simulink model "ctrl_custom"  (R2016b)
settings: Solver=ode3  StartTime=0.0  StopTime=inf  FixedStep=0.01  RelTol=1e-3  EnableMultiTasking=on
undefined symbols (not defined in the file): C, D, DiscIntNeverNeededParam, eps_c, epsilon, hd, hd2, I_s, k_cc, K_omega, K_q1f, K_q1r, K_q2f, K_q2r, K_q3f, K_q3r, K_q4f, K_q4r, K_q5f, K_q5r, K_q6f, K_q6r, K_T1f, K_T1r, K_T2f, K_T2r, K_T3f, K_T3r, K_T4f, K_T4r, K_T5f, K_T5r, K_T6f, K_T6r, Kp, Max_Acceleration, Max_rotation, Max_thrust, Min_thrust, n_c, n_max, p_cc, pwm_thr1_backward, pwm_thr1_forward, pwm_thr2_backward, pwm_thr2_forward, pwm_thr3_backward, pwm_thr3_forward, pwm_thr4_backward, pwm_thr4_forward, pwm_thr5_backward, pwm_thr5_forward, pwm_thr6_backward, pwm_thr6_forward, Q_f0, Q_max, r_cc, Rho, Thruster
libraries: dspmtrx3 x9, marine_gnc x9, simulink x7, simulink_extras x3
(part 3 of 6)

== system ctrl_custom/Initialization of parameters/Control Gains ==
  Create Diagonal Matrix : dspmtrx3/Create Diagonal Matrix
  Create Diagonal Matrix1 : dspmtrx3/Create Diagonal Matrix
  Create Diagonal Matrix2 : dspmtrx3/Create Diagonal Matrix
  K_d_psi : S-Function  Priority=7  FunctionName=NIVeriStandIO  Parameters=width dtype portnum stime stype btype  SFunctionDeploymentMode=off  EnableBusSupport=off  mask(NI VeriStand Inport){portnum=7, width=-1, stime=-1, dtype=auto, stype=auto, btype=1}
      mask prompts: portnum "Port number:"; width "Port dimensions (-1 for dynamically sized):"; stime "Sample time (-1 for inherited):"; dtype "Data type:"; stype "Signal type:"; btype "Block type:"
      mask help: Use this inport on any level of nested subsystems to allow NI VeriStand software to map signals to it.
      mask init:
      | NIVeriStandIO_init;
      settings: CopyFcn=NIVeriStand_MDL_functions('', 'IO_copy');  DeleteFcn=NIVeriStand_MDL_functions('', 'IO_delete');  MoveFcn=set_param(gcb, 'Mask', 'on');
      mask Callback portnum: NIVeriStand_MDL_functions('', 'IO_setportnum');
      mask TypeOptions dtype: auto | double | single | int8 | uint8 | int16 | uint16 | int32 | uint32 | boolean
      mask Callback dtype: NIVeriStand_MDL_functions('', 'IO_booleansignal');
      mask TypeOptions stype: auto | real | complex
      mask Display:
      | patch([-x x], [-y y], [.90980 .81960 .32156]);
      | plot([xrad -x x xrad], [yrad -y y yrad]);
      | fprintf('NI In%d', portnum);
  K_d_x : S-Function  Priority=8  FunctionName=NIVeriStandIO  Parameters=width dtype portnum stime stype btype  SFunctionDeploymentMode=off  EnableBusSupport=off  mask(NI VeriStand Inport){portnum=8, width=-1, stime=-1, dtype=auto, stype=auto, btype=1}
      mask prompts: portnum "Port number:"; width "Port dimensions (-1 for dynamically sized):"; stime "Sample time (-1 for inherited):"; dtype "Data type:"; stype "Signal type:"; btype "Block type:"
      mask help: Use this inport on any level of nested subsystems to allow NI VeriStand software to map signals to it.
      mask init:
      | NIVeriStandIO_init;
      settings: CopyFcn=NIVeriStand_MDL_functions('', 'IO_copy');  DeleteFcn=NIVeriStand_MDL_functions('', 'IO_delete');  MoveFcn=set_param(gcb, 'Mask', 'on');
      mask Callback portnum: NIVeriStand_MDL_functions('', 'IO_setportnum');
      mask TypeOptions dtype: auto | double | single | int8 | uint8 | int16 | uint16 | int32 | uint32 | boolean
      mask Callback dtype: NIVeriStand_MDL_functions('', 'IO_booleansignal');
      mask TypeOptions stype: auto | real | complex
      mask Display:
      | patch([-x x], [-y y], [.90980 .81960 .32156]);
      | plot([xrad -x x xrad], [yrad -y y yrad]);
      | fprintf('NI In%d', portnum);
  K_d_y : S-Function  Priority=9  FunctionName=NIVeriStandIO  Parameters=width dtype portnum stime stype btype  SFunctionDeploymentMode=off  EnableBusSupport=off  mask(NI VeriStand Inport){portnum=9, width=-1, stime=-1, dtype=auto, stype=auto, btype=1}
      mask prompts: portnum "Port number:"; width "Port dimensions (-1 for dynamically sized):"; stime "Sample time (-1 for inherited):"; dtype "Data type:"; stype "Signal type:"; btype "Block type:"
      mask help: Use this inport on any level of nested subsystems to allow NI VeriStand software to map signals to it.
      mask init:
      | NIVeriStandIO_init;
      settings: CopyFcn=NIVeriStand_MDL_functions('', 'IO_copy');  DeleteFcn=NIVeriStand_MDL_functions('', 'IO_delete');  MoveFcn=set_param(gcb, 'Mask', 'on');
      mask Callback portnum: NIVeriStand_MDL_functions('', 'IO_setportnum');
      mask TypeOptions dtype: auto | double | single | int8 | uint8 | int16 | uint16 | int32 | uint32 | boolean
      mask Callback dtype: NIVeriStand_MDL_functions('', 'IO_booleansignal');
      mask TypeOptions stype: auto | real | complex
      mask Display:
      | patch([-x x], [-y y], [.90980 .81960 .32156]);
      | plot([xrad -x x xrad], [yrad -y y yrad]);
      | fprintf('NI In%d', portnum);
  K_i_psi : S-Function  Priority=4  FunctionName=NIVeriStandIO  Parameters=width dtype portnum stime stype btype  SFunctionDeploymentMode=off  EnableBusSupport=off  mask(NI VeriStand Inport){portnum=4, width=-1, stime=-1, dtype=auto, stype=auto, btype=1}
      mask prompts: portnum "Port number:"; width "Port dimensions (-1 for dynamically sized):"; stime "Sample time (-1 for inherited):"; dtype "Data type:"; stype "Signal type:"; btype "Block type:"
      mask help: Use this inport on any level of nested subsystems to allow NI VeriStand software to map signals to it.
      mask init:
      | NIVeriStandIO_init;
      settings: CopyFcn=NIVeriStand_MDL_functions('', 'IO_copy');  DeleteFcn=NIVeriStand_MDL_functions('', 'IO_delete');  MoveFcn=set_param(gcb, 'Mask', 'on');
      mask Callback portnum: NIVeriStand_MDL_functions('', 'IO_setportnum');
      mask TypeOptions dtype: auto | double | single | int8 | uint8 | int16 | uint16 | int32 | uint32 | boolean
      mask Callback dtype: NIVeriStand_MDL_functions('', 'IO_booleansignal');
      mask TypeOptions stype: auto | real | complex
      mask Display:
      | patch([-x x], [-y y], [.90980 .81960 .32156]);
      | plot([xrad -x x xrad], [yrad -y y yrad]);
      | fprintf('NI In%d', portnum);
  K_i_x : S-Function  Priority=5  FunctionName=NIVeriStandIO  Parameters=width dtype portnum stime stype btype  SFunctionDeploymentMode=off  EnableBusSupport=off  mask(NI VeriStand Inport){portnum=5, width=-1, stime=-1, dtype=auto, stype=auto, btype=1}
      mask prompts: portnum "Port number:"; width "Port dimensions (-1 for dynamically sized):"; stime "Sample time (-1 for inherited):"; dtype "Data type:"; stype "Signal type:"; btype "Block type:"
      mask help: Use this inport on any level of nested subsystems to allow NI VeriStand software to map signals to it.
      mask init:
      | NIVeriStandIO_init;
      settings: CopyFcn=NIVeriStand_MDL_functions('', 'IO_copy');  DeleteFcn=NIVeriStand_MDL_functions('', 'IO_delete');  MoveFcn=set_param(gcb, 'Mask', 'on');
      mask Callback portnum: NIVeriStand_MDL_functions('', 'IO_setportnum');
      mask TypeOptions dtype: auto | double | single | int8 | uint8 | int16 | uint16 | int32 | uint32 | boolean
      mask Callback dtype: NIVeriStand_MDL_functions('', 'IO_booleansignal');
      mask TypeOptions stype: auto | real | complex
      mask Display:
      | patch([-x x], [-y y], [.90980 .81960 .32156]);
      | plot([xrad -x x xrad], [yrad -y y yrad]);
      | fprintf('NI In%d', portnum);
  K_i_y : S-Function  Priority=6  FunctionName=NIVeriStandIO  Parameters=width dtype portnum stime stype btype  SFunctionDeploymentMode=off  EnableBusSupport=off  mask(NI VeriStand Inport){portnum=6, width=-1, stime=-1, dtype=auto, stype=auto, btype=1}
      mask prompts: portnum "Port number:"; width "Port dimensions (-1 for dynamically sized):"; stime "Sample time (-1 for inherited):"; dtype "Data type:"; stype "Signal type:"; btype "Block type:"
      mask help: Use this inport on any level of nested subsystems to allow NI VeriStand software to map signals to it.
      mask init:
      | NIVeriStandIO_init;
      settings: CopyFcn=NIVeriStand_MDL_functions('', 'IO_copy');  DeleteFcn=NIVeriStand_MDL_functions('', 'IO_delete');  MoveFcn=set_param(gcb, 'Mask', 'on');
      mask Callback portnum: NIVeriStand_MDL_functions('', 'IO_setportnum');
      mask TypeOptions dtype: auto | double | single | int8 | uint8 | int16 | uint16 | int32 | uint32 | boolean
      mask Callback dtype: NIVeriStand_MDL_functions('', 'IO_booleansignal');
      mask TypeOptions stype: auto | real | complex
      mask Display:
      | patch([-x x], [-y y], [.90980 .81960 .32156]);
      | plot([xrad -x x xrad], [yrad -y y yrad]);
      | fprintf('NI In%d', portnum);
  K_p_psi : S-Function  Priority=3  FunctionName=NIVeriStandIO  Parameters=width dtype portnum stime stype btype  SFunctionDeploymentMode=off  EnableBusSupport=off  mask(NI VeriStand Inport){portnum=3, width=-1, stime=-1, dtype=auto, stype=auto, btype=1}
      mask prompts: portnum "Port number:"; width "Port dimensions (-1 for dynamically sized):"; stime "Sample time (-1 for inherited):"; dtype "Data type:"; stype "Signal type:"; btype "Block type:"
      mask help: Use this inport on any level of nested subsystems to allow NI VeriStand software to map signals to it.
      mask init:
      | NIVeriStandIO_init;
      settings: CopyFcn=NIVeriStand_MDL_functions('', 'IO_copy');  DeleteFcn=NIVeriStand_MDL_functions('', 'IO_delete');  MoveFcn=set_param(gcb, 'Mask', 'on');
      mask Callback portnum: NIVeriStand_MDL_functions('', 'IO_setportnum');
      mask TypeOptions dtype: auto | double | single | int8 | uint8 | int16 | uint16 | int32 | uint32 | boolean
      mask Callback dtype: NIVeriStand_MDL_functions('', 'IO_booleansignal');
      mask TypeOptions stype: auto | real | complex
      mask Display:
      | patch([-x x], [-y y], [.90980 .81960 .32156]);
      | plot([xrad -x x xrad], [yrad -y y yrad]);
      | fprintf('NI In%d', portnum);
  K_p_x : S-Function  Priority=1  FunctionName=NIVeriStandIO  Parameters=width dtype portnum stime stype btype  SFunctionDeploymentMode=off  EnableBusSupport=off  mask(NI VeriStand Inport){portnum=1, width=-1, stime=-1, dtype=auto, stype=auto, btype=1}
      mask prompts: portnum "Port number:"; width "Port dimensions (-1 for dynamically sized):"; stime "Sample time (-1 for inherited):"; dtype "Data type:"; stype "Signal type:"; btype "Block type:"
      mask help: Use this inport on any level of nested subsystems to allow NI VeriStand software to map signals to it.
      mask init:
      | NIVeriStandIO_init;
      settings: CopyFcn=NIVeriStand_MDL_functions('', 'IO_copy');  DeleteFcn=NIVeriStand_MDL_functions('', 'IO_delete');  MoveFcn=set_param(gcb, 'Mask', 'on');
      mask Callback portnum: NIVeriStand_MDL_functions('', 'IO_setportnum');
      mask TypeOptions dtype: auto | double | single | int8 | uint8 | int16 | uint16 | int32 | uint32 | boolean
      mask Callback dtype: NIVeriStand_MDL_functions('', 'IO_booleansignal');
      mask TypeOptions stype: auto | real | complex
      mask Display:
      | patch([-x x], [-y y], [.90980 .81960 .32156]);
      | plot([xrad -x x xrad], [yrad -y y yrad]);
      | fprintf('NI In%d', portnum);
  K_p_y : S-Function  Priority=2  FunctionName=NIVeriStandIO  Parameters=width dtype portnum stime stype btype  SFunctionDeploymentMode=off  EnableBusSupport=off  mask(NI VeriStand Inport){portnum=2, width=-1, stime=-1, dtype=auto, stype=auto, btype=1}
      mask prompts: portnum "Port number:"; width "Port dimensions (-1 for dynamically sized):"; stime "Sample time (-1 for inherited):"; dtype "Data type:"; stype "Signal type:"; btype "Block type:"
      mask help: Use this inport on any level of nested subsystems to allow NI VeriStand software to map signals to it.
      mask init:
      | NIVeriStandIO_init;
      settings: CopyFcn=NIVeriStand_MDL_functions('', 'IO_copy');  DeleteFcn=NIVeriStand_MDL_functions('', 'IO_delete');  MoveFcn=set_param(gcb, 'Mask', 'on');
      mask Callback portnum: NIVeriStand_MDL_functions('', 'IO_setportnum');
      mask TypeOptions dtype: auto | double | single | int8 | uint8 | int16 | uint16 | int32 | uint32 | boolean
      mask Callback dtype: NIVeriStand_MDL_functions('', 'IO_booleansignal');
      mask TypeOptions stype: auto | real | complex
      mask Display:
      | patch([-x x], [-y y], [.90980 .81960 .32156]);
      | plot([xrad -x x xrad], [yrad -y y yrad]);
      | fprintf('NI In%d', portnum);
  Mux1 : Mux  Inputs=3
  Mux2 : Mux  Inputs=3
  Mux3 : Mux  Inputs=3
  tag scope: K_d=global, K_i=global, K_p=global, Kd_psi=global, Ki_psi=global, Kp_psi=global
  wires:
  K_p_x/1 -> Mux1/1
  K_p_psi/1 -> [Kp_psi], Mux1/3
  K_p_y/1 -> Mux1/2
  Mux1/1 -> Create Diagonal Matrix/1
  Create Diagonal Matrix/1 -> [K_p]
  Mux2/1 -> Create Diagonal Matrix1/1
  K_d_x/1 -> Mux3/1
  K_d_psi/1 -> [Kd_psi], Mux3/3
  K_d_y/1 -> Mux3/2
  Mux3/1 -> Create Diagonal Matrix2/1
  Create Diagonal Matrix1/1 -> [K_i]
  Create Diagonal Matrix2/1 -> [K_d]
  K_i_x/1 -> Mux2/1
  K_i_y/1 -> Mux2/2
  K_i_psi/1 -> [Ki_psi], Mux2/3

== system ctrl_custom/Initialization of parameters/Guidance Gains ==
  Create Diagonal Matrix3 : dspmtrx3/Create Diagonal Matrix
  Create Diagonal Matrix4 : dspmtrx3/Create Diagonal Matrix
  Create Diagonal Matrix5 : dspmtrx3/Create Diagonal Matrix
  MATLAB Function : MATLAB Function  TreatAsAtomicUnit=on
  MATLAB Function1 : MATLAB Function  TreatAsAtomicUnit=on
  MATLAB Function2 : MATLAB Function  TreatAsAtomicUnit=on
  Mux3 : Mux  Inputs=3
  Mux4 : Mux  Inputs=3
  Mux5 : Mux  Inputs=3
  T_psi : S-Function  Priority=7  FunctionName=NIVeriStandIO  Parameters=width dtype portnum stime stype btype  SFunctionDeploymentMode=off  EnableBusSupport=off  mask(NI VeriStand Inport){portnum=7, width=-1, stime=-1, dtype=auto, stype=auto, btype=1}
      mask prompts: portnum "Port number:"; width "Port dimensions (-1 for dynamically sized):"; stime "Sample time (-1 for inherited):"; dtype "Data type:"; stype "Signal type:"; btype "Block type:"
      mask help: Use this inport on any level of nested subsystems to allow NI VeriStand software to map signals to it.
      mask init:
      | NIVeriStandIO_init;
      settings: CopyFcn=NIVeriStand_MDL_functions('', 'IO_copy');  DeleteFcn=NIVeriStand_MDL_functions('', 'IO_delete');  MoveFcn=set_param(gcb, 'Mask', 'on');
      mask Callback portnum: NIVeriStand_MDL_functions('', 'IO_setportnum');
      mask TypeOptions dtype: auto | double | single | int8 | uint8 | int16 | uint16 | int32 | uint32 | boolean
      mask Callback dtype: NIVeriStand_MDL_functions('', 'IO_booleansignal');
      mask TypeOptions stype: auto | real | complex
      mask Display:
      | patch([-x x], [-y y], [.90980 .81960 .32156]);
      | plot([xrad -x x xrad], [yrad -y y yrad]);
      | fprintf('NI In%d', portnum);
  T_x : S-Function  Priority=8  FunctionName=NIVeriStandIO  Parameters=width dtype portnum stime stype btype  SFunctionDeploymentMode=off  EnableBusSupport=off  mask(NI VeriStand Inport){portnum=8, width=-1, stime=-1, dtype=auto, stype=auto, btype=1}
      mask prompts: portnum "Port number:"; width "Port dimensions (-1 for dynamically sized):"; stime "Sample time (-1 for inherited):"; dtype "Data type:"; stype "Signal type:"; btype "Block type:"
      mask help: Use this inport on any level of nested subsystems to allow NI VeriStand software to map signals to it.
      mask init:
      | NIVeriStandIO_init;
      settings: CopyFcn=NIVeriStand_MDL_functions('', 'IO_copy');  DeleteFcn=NIVeriStand_MDL_functions('', 'IO_delete');  MoveFcn=set_param(gcb, 'Mask', 'on');
      mask Callback portnum: NIVeriStand_MDL_functions('', 'IO_setportnum');
      mask TypeOptions dtype: auto | double | single | int8 | uint8 | int16 | uint16 | int32 | uint32 | boolean
      mask Callback dtype: NIVeriStand_MDL_functions('', 'IO_booleansignal');
      mask TypeOptions stype: auto | real | complex
      mask Display:
      | patch([-x x], [-y y], [.90980 .81960 .32156]);
      | plot([xrad -x x xrad], [yrad -y y yrad]);
      | fprintf('NI In%d', portnum);
  T_y : S-Function  Priority=9  FunctionName=NIVeriStandIO  Parameters=width dtype portnum stime stype btype  SFunctionDeploymentMode=off  EnableBusSupport=off  mask(NI VeriStand Inport){portnum=9, width=-1, stime=-1, dtype=auto, stype=auto, btype=1}
      mask prompts: portnum "Port number:"; width "Port dimensions (-1 for dynamically sized):"; stime "Sample time (-1 for inherited):"; dtype "Data type:"; stype "Signal type:"; btype "Block type:"
      mask help: Use this inport on any level of nested subsystems to allow NI VeriStand software to map signals to it.
      mask init:
      | NIVeriStandIO_init;
      settings: CopyFcn=NIVeriStand_MDL_functions('', 'IO_copy');  DeleteFcn=NIVeriStand_MDL_functions('', 'IO_delete');  MoveFcn=set_param(gcb, 'Mask', 'on');
      mask Callback portnum: NIVeriStand_MDL_functions('', 'IO_setportnum');
      mask TypeOptions dtype: auto | double | single | int8 | uint8 | int16 | uint16 | int32 | uint32 | boolean
      mask Callback dtype: NIVeriStand_MDL_functions('', 'IO_booleansignal');
      mask TypeOptions stype: auto | real | complex
      mask Display:
      | patch([-x x], [-y y], [.90980 .81960 .32156]);
      | plot([xrad -x x xrad], [yrad -y y yrad]);
      | fprintf('NI In%d', portnum);
  w_psi : S-Function  Priority=3  FunctionName=NIVeriStandIO  Parameters=width dtype portnum stime stype btype  SFunctionDeploymentMode=off  EnableBusSupport=off  mask(NI VeriStand Inport){portnum=3, width=-1, stime=-1, dtype=auto, stype=auto, btype=1}
      mask prompts: portnum "Port number:"; width "Port dimensions (-1 for dynamically sized):"; stime "Sample time (-1 for inherited):"; dtype "Data type:"; stype "Signal type:"; btype "Block type:"
      mask help: Use this inport on any level of nested subsystems to allow NI VeriStand software to map signals to it.
      mask init:
      | NIVeriStandIO_init;
      settings: CopyFcn=NIVeriStand_MDL_functions('', 'IO_copy');  DeleteFcn=NIVeriStand_MDL_functions('', 'IO_delete');  MoveFcn=set_param(gcb, 'Mask', 'on');
      mask Callback portnum: NIVeriStand_MDL_functions('', 'IO_setportnum');
      mask TypeOptions dtype: auto | double | single | int8 | uint8 | int16 | uint16 | int32 | uint32 | boolean
      mask Callback dtype: NIVeriStand_MDL_functions('', 'IO_booleansignal');
      mask TypeOptions stype: auto | real | complex
      mask Display:
      | patch([-x x], [-y y], [.90980 .81960 .32156]);
      | plot([xrad -x x xrad], [yrad -y y yrad]);
      | fprintf('NI In%d', portnum);
  w_x : S-Function  Priority=1  FunctionName=NIVeriStandIO  Parameters=width dtype portnum stime stype btype  SFunctionDeploymentMode=off  EnableBusSupport=off  mask(NI VeriStand Inport){portnum=1, width=-1, stime=-1, dtype=auto, stype=auto, btype=1}
      mask prompts: portnum "Port number:"; width "Port dimensions (-1 for dynamically sized):"; stime "Sample time (-1 for inherited):"; dtype "Data type:"; stype "Signal type:"; btype "Block type:"
      mask help: Use this inport on any level of nested subsystems to allow NI VeriStand software to map signals to it.
      mask init:
      | NIVeriStandIO_init;
      settings: CopyFcn=NIVeriStand_MDL_functions('', 'IO_copy');  DeleteFcn=NIVeriStand_MDL_functions('', 'IO_delete');  MoveFcn=set_param(gcb, 'Mask', 'on');
      mask Callback portnum: NIVeriStand_MDL_functions('', 'IO_setportnum');
      mask TypeOptions dtype: auto | double | single | int8 | uint8 | int16 | uint16 | int32 | uint32 | boolean
      mask Callback dtype: NIVeriStand_MDL_functions('', 'IO_booleansignal');
      mask TypeOptions stype: auto | real | complex
      mask Display:
      | patch([-x x], [-y y], [.90980 .81960 .32156]);
      | plot([xrad -x x xrad], [yrad -y y yrad]);
      | fprintf('NI In%d', portnum);
  w_y : S-Function  Priority=2  FunctionName=NIVeriStandIO  Parameters=width dtype portnum stime stype btype  SFunctionDeploymentMode=off  EnableBusSupport=off  mask(NI VeriStand Inport){portnum=2, width=-1, stime=-1, dtype=auto, stype=auto, btype=1}
      mask prompts: portnum "Port number:"; width "Port dimensions (-1 for dynamically sized):"; stime "Sample time (-1 for inherited):"; dtype "Data type:"; stype "Signal type:"; btype "Block type:"
      mask help: Use this inport on any level of nested subsystems to allow NI VeriStand software to map signals to it.
      mask init:
      | NIVeriStandIO_init;
      settings: CopyFcn=NIVeriStand_MDL_functions('', 'IO_copy');  DeleteFcn=NIVeriStand_MDL_functions('', 'IO_delete');  MoveFcn=set_param(gcb, 'Mask', 'on');
      mask Callback portnum: NIVeriStand_MDL_functions('', 'IO_setportnum');
      mask TypeOptions dtype: auto | double | single | int8 | uint8 | int16 | uint16 | int32 | uint32 | boolean
      mask Callback dtype: NIVeriStand_MDL_functions('', 'IO_booleansignal');
      mask TypeOptions stype: auto | real | complex
      mask Display:
      | patch([-x x], [-y y], [.90980 .81960 .32156]);
      | plot([xrad -x x xrad], [yrad -y y yrad]);
      | fprintf('NI In%d', portnum);
  zeta_psi : S-Function  Priority=4  FunctionName=NIVeriStandIO  Parameters=width dtype portnum stime stype btype  SFunctionDeploymentMode=off  EnableBusSupport=off  mask(NI VeriStand Inport){portnum=4, width=-1, stime=-1, dtype=auto, stype=auto, btype=1}
      mask prompts: portnum "Port number:"; width "Port dimensions (-1 for dynamically sized):"; stime "Sample time (-1 for inherited):"; dtype "Data type:"; stype "Signal type:"; btype "Block type:"
      mask help: Use this inport on any level of nested subsystems to allow NI VeriStand software to map signals to it.
      mask init:
      | NIVeriStandIO_init;
      settings: CopyFcn=NIVeriStand_MDL_functions('', 'IO_copy');  DeleteFcn=NIVeriStand_MDL_functions('', 'IO_delete');  MoveFcn=set_param(gcb, 'Mask', 'on');
      mask Callback portnum: NIVeriStand_MDL_functions('', 'IO_setportnum');
      mask TypeOptions dtype: auto | double | single | int8 | uint8 | int16 | uint16 | int32 | uint32 | boolean
      mask Callback dtype: NIVeriStand_MDL_functions('', 'IO_booleansignal');
      mask TypeOptions stype: auto | real | complex
      mask Display:
      | patch([-x x], [-y y], [.90980 .81960 .32156]);
      | plot([xrad -x x xrad], [yrad -y y yrad]);
      | fprintf('NI In%d', portnum);
  zeta_x : S-Function  Priority=5  FunctionName=NIVeriStandIO  Parameters=width dtype portnum stime stype btype  SFunctionDeploymentMode=off  EnableBusSupport=off  mask(NI VeriStand Inport){portnum=5, width=-1, stime=-1, dtype=auto, stype=auto, btype=1}
      mask prompts: portnum "Port number:"; width "Port dimensions (-1 for dynamically sized):"; stime "Sample time (-1 for inherited):"; dtype "Data type:"; stype "Signal type:"; btype "Block type:"
      mask help: Use this inport on any level of nested subsystems to allow NI VeriStand software to map signals to it.
      mask init:
      | NIVeriStandIO_init;
      settings: CopyFcn=NIVeriStand_MDL_functions('', 'IO_copy');  DeleteFcn=NIVeriStand_MDL_functions('', 'IO_delete');  MoveFcn=set_param(gcb, 'Mask', 'on');
      mask Callback portnum: NIVeriStand_MDL_functions('', 'IO_setportnum');
      mask TypeOptions dtype: auto | double | single | int8 | uint8 | int16 | uint16 | int32 | uint32 | boolean
      mask Callback dtype: NIVeriStand_MDL_functions('', 'IO_booleansignal');
      mask TypeOptions stype: auto | real | complex
      mask Display:
      | patch([-x x], [-y y], [.90980 .81960 .32156]);
      | plot([xrad -x x xrad], [yrad -y y yrad]);
      | fprintf('NI In%d', portnum);
  zeta_y : S-Function  Priority=6  FunctionName=NIVeriStandIO  Parameters=width dtype portnum stime stype btype  SFunctionDeploymentMode=off  EnableBusSupport=off  mask(NI VeriStand Inport){portnum=6, width=-1, stime=-1, dtype=auto, stype=auto, btype=1}
      mask prompts: portnum "Port number:"; width "Port dimensions (-1 for dynamically sized):"; stime "Sample time (-1 for inherited):"; dtype "Data type:"; stype "Signal type:"; btype "Block type:"
      mask help: Use this inport on any level of nested subsystems to allow NI VeriStand software to map signals to it.
      mask init:
      | NIVeriStandIO_init;
      settings: CopyFcn=NIVeriStand_MDL_functions('', 'IO_copy');  DeleteFcn=NIVeriStand_MDL_functions('', 'IO_delete');  MoveFcn=set_param(gcb, 'Mask', 'on');
      mask Callback portnum: NIVeriStand_MDL_functions('', 'IO_setportnum');
      mask TypeOptions dtype: auto | double | single | int8 | uint8 | int16 | uint16 | int32 | uint32 | boolean
      mask Callback dtype: NIVeriStand_MDL_functions('', 'IO_booleansignal');
      mask TypeOptions stype: auto | real | complex
      mask Display:
      | patch([-x x], [-y y], [.90980 .81960 .32156]);
      | plot([xrad -x x xrad], [yrad -y y yrad]);
      | fprintf('NI In%d', portnum);
  tag scope: Af=global, omega=global, zeta=global
  wires:
  w_x/1 -> Mux3/1
  w_psi/1 -> Mux3/3
  w_y/1 -> Mux3/2
  Mux3/1 -> Create Diagonal Matrix3/1
  Create Diagonal Matrix3/1 -> [omega]
  Mux4/1 -> Create Diagonal Matrix4/1
  T_x/1 -> MATLAB Function/1(T_x)
  T_psi/1 -> MATLAB Function2/1(T_psi)
  T_y/1 -> MATLAB Function1/1(T_y)
  Mux5/1 -> Create Diagonal Matrix5/1
  Create Diagonal Matrix4/1 -> [zeta]
  Create Diagonal Matrix5/1 -> [Af]
  zeta_x/1 -> Mux4/1
  zeta_y/1 -> Mux4/2
  zeta_psi/1 -> Mux4/3
  MATLAB Function/1(y) -> Mux5/1
  MATLAB Function1/1(y) -> Mux5/2
  MATLAB Function2/1(y) -> Mux5/3

== system ctrl_custom/Initialization of parameters/Observer Gains ==
  Constant : Constant  Value=50
  Constant1 : Constant  Value=50
  Constant2 : Constant  Value=50
  Constant{3..8} (6 alike) : Constant
  Create Diagonal Matrix : dspmtrx3/Create Diagonal Matrix
  Create Diagonal Matrix1 : dspmtrx3/Create Diagonal Matrix
  Create Diagonal Matrix2 : dspmtrx3/Create Diagonal Matrix
  Mux1 : Mux  Inputs=3
  Mux2 : Mux  Inputs=3
  Mux3 : Mux  Inputs=3
  tag scope: K_2=global, K_3=global, K_4=global
  wires:
  Constant/1 -> Mux1/1
  Constant2/1 -> Mux1/3
  Constant1/1 -> Mux1/2
  Mux1/1 -> Create Diagonal Matrix/1
  Create Diagonal Matrix/1 -> [K_2]
  Constant3/1 -> Mux2/1
  Constant5/1 -> Mux2/3
  Constant4/1 -> Mux2/2
  Mux2/1 -> Create Diagonal Matrix1/1
  Constant8/1 -> Mux3/3
  Constant7/1 -> Mux3/2
  Mux3/1 -> Create Diagonal Matrix2/1
  Create Diagonal Matrix1/1 -> [K_3]
  Create Diagonal Matrix2/1 -> [K_4]
  Constant6/1 -> Mux3/1

== system ctrl_custom/Nonlinear Passisve Observer/Transpose Rotation Matrix ==
  psi : Inport
  y_tilde : Inport  Port=2
  Mux : Mux  Inputs=2
  Mux1 : Mux  Inputs=3
  Row1 : Fcn  Expr=cos(u(1))*u(2)+sin(u(1))*u(3)
  Row2 : Fcn  Expr=-sin(u(1))*u(2)+cos(u(1))*u(3)
  Row3 : Fcn  Expr=u(4)
  R(psi)'*y_tilde : Outport
  wires:
  Mux/1 -> Row3/1, Row2/1, Row1/1
  Row1/1 -> Mux1/1
  Row2/1 -> Mux1/2
  Row3/1 -> Mux1/3
  Mux1/1 -> R(psi)'*y_tilde/1
  psi/1 -> Mux/1
  y_tilde/1 -> Mux/2

== system ctrl_custom/Nonlinear Passisve Observer/Transpose Rotation matrix ==
  psi : Inport
  b_hat : Inport  Port=2
  Mux : Mux  Inputs=2
  Mux1 : Mux  Inputs=3
  Row1 : Fcn  Expr=cos(u(1))*u(2)+sin(u(1))*u(3)
  Row2 : Fcn  Expr=-sin(u(1))*u(2)+cos(u(1))*u(3)
  Row3 : Fcn  Expr=u(4)
  R(psi)'*b_hat : Outport
  wires:
  Mux/1 -> Row3/1, Row2/1, Row1/1
  Row1/1 -> Mux1/1
  Row2/1 -> Mux1/2
  Row3/1 -> Mux1/3
  Mux1/1 -> R(psi)'*b_hat/1
  psi/1 -> Mux/1
  b_hat/1 -> Mux/2

== system ctrl_custom/Observer output /b_hat output ==
  b_hat : Inport
  Demux : Demux  Outputs=3
  b_psi_hat : S-Function  Priority=3  FunctionName=NIVeriStandIO  Parameters=width dtype portnum stime stype btype  SFunctionDeploymentMode=off  EnableBusSupport=off  mask(NI VeriStand Outport){portnum=3, width=-1, stime=-1, dtype=auto, stype=auto, btype=0}
      mask prompts: portnum "Port number:"; width "Port dimensions (-1 for dynamically sized):"; stime "Sample time (-1 for inherited):"; dtype "Data type:"; stype "Signal type:"; btype "Block type:"
      mask help: Use this outport on any level of nested subsystems to allow NI VeriStand software to map signals to it.
      mask init:
      | NIVeriStandIO_init;
      settings: CopyFcn=NIVeriStand_MDL_functions('', 'IO_copy');  DeleteFcn=NIVeriStand_MDL_functions('', 'IO_delete');  MoveFcn=set_param(gcb, 'Mask', 'on');
      mask Callback portnum: NIVeriStand_MDL_functions('', 'IO_setportnum');
      mask TypeOptions dtype: auto | double | single | int8 | uint8 | int16 | uint16 | int32 | uint32 | boolean
      mask Callback dtype: NIVeriStand_MDL_functions('', 'IO_booleansignal');
      mask TypeOptions stype: auto | real | complex
      mask Display:
      | patch([-x x], [-y y], [.90980 .81960 .32156]);
      | plot([xrad -x x xrad], [yrad -y y yrad]);
      | fprintf('NI Out%d', portnum);
  b_x_hat : S-Function  Priority=1  FunctionName=NIVeriStandIO  Parameters=width dtype portnum stime stype btype  SFunctionDeploymentMode=off  EnableBusSupport=off  mask(NI VeriStand Outport){portnum=1, width=-1, stime=-1, dtype=auto, stype=auto, btype=0}
      mask prompts: portnum "Port number:"; width "Port dimensions (-1 for dynamically sized):"; stime "Sample time (-1 for inherited):"; dtype "Data type:"; stype "Signal type:"; btype "Block type:"
      mask help: Use this outport on any level of nested subsystems to allow NI VeriStand software to map signals to it.
      mask init:
      | NIVeriStandIO_init;
      settings: CopyFcn=NIVeriStand_MDL_functions('', 'IO_copy');  DeleteFcn=NIVeriStand_MDL_functions('', 'IO_delete');  MoveFcn=set_param(gcb, 'Mask', 'on');
      mask Callback portnum: NIVeriStand_MDL_functions('', 'IO_setportnum');
      mask TypeOptions dtype: auto | double | single | int8 | uint8 | int16 | uint16 | int32 | uint32 | boolean
      mask Callback dtype: NIVeriStand_MDL_functions('', 'IO_booleansignal');
      mask TypeOptions stype: auto | real | complex
      mask Display:
      | patch([-x x], [-y y], [.90980 .81960 .32156]);
      | plot([xrad -x x xrad], [yrad -y y yrad]);
      | fprintf('NI Out%d', portnum);
  b_y_hat : S-Function  Priority=2  FunctionName=NIVeriStandIO  Parameters=width dtype portnum stime stype btype  SFunctionDeploymentMode=off  EnableBusSupport=off  mask(NI VeriStand Outport){portnum=2, width=-1, stime=-1, dtype=auto, stype=auto, btype=0}
      mask prompts: portnum "Port number:"; width "Port dimensions (-1 for dynamically sized):"; stime "Sample time (-1 for inherited):"; dtype "Data type:"; stype "Signal type:"; btype "Block type:"
      mask help: Use this outport on any level of nested subsystems to allow NI VeriStand software to map signals to it.
      mask init:
      | NIVeriStandIO_init;
      settings: CopyFcn=NIVeriStand_MDL_functions('', 'IO_copy');  DeleteFcn=NIVeriStand_MDL_functions('', 'IO_delete');  MoveFcn=set_param(gcb, 'Mask', 'on');
      mask Callback portnum: NIVeriStand_MDL_functions('', 'IO_setportnum');
      mask TypeOptions dtype: auto | double | single | int8 | uint8 | int16 | uint16 | int32 | uint32 | boolean
      mask Callback dtype: NIVeriStand_MDL_functions('', 'IO_booleansignal');
      mask TypeOptions stype: auto | real | complex
      mask Display:
      | patch([-x x], [-y y], [.90980 .81960 .32156]);
      | plot([xrad -x x xrad], [yrad -y y yrad]);
      | fprintf('NI Out%d', portnum);
  wires:
  Demux/1 -> b_x_hat/1
  Demux/2 -> b_y_hat/1
  Demux/3 -> b_psi_hat/1
  b_hat/1 -> Demux/1

== system ctrl_custom/Observer output /eta_hat output ==
  eta-_hat : Inport
  Demux : Demux  Outputs=3
  psi_hat : S-Function  Priority=3  FunctionName=NIVeriStandIO  Parameters=width dtype portnum stime stype btype  SFunctionDeploymentMode=off  EnableBusSupport=off  mask(NI VeriStand Outport){portnum=3, width=-1, stime=-1, dtype=auto, stype=auto, btype=0}
      mask prompts: portnum "Port number:"; width "Port dimensions (-1 for dynamically sized):"; stime "Sample time (-1 for inherited):"; dtype "Data type:"; stype "Signal type:"; btype "Block type:"
      mask help: Use this outport on any level of nested subsystems to allow NI VeriStand software to map signals to it.
      mask init:
      | NIVeriStandIO_init;
      settings: CopyFcn=NIVeriStand_MDL_functions('', 'IO_copy');  DeleteFcn=NIVeriStand_MDL_functions('', 'IO_delete');  MoveFcn=set_param(gcb, 'Mask', 'on');
      mask Callback portnum: NIVeriStand_MDL_functions('', 'IO_setportnum');
      mask TypeOptions dtype: auto | double | single | int8 | uint8 | int16 | uint16 | int32 | uint32 | boolean
      mask Callback dtype: NIVeriStand_MDL_functions('', 'IO_booleansignal');
      mask TypeOptions stype: auto | real | complex
      mask Display:
      | patch([-x x], [-y y], [.90980 .81960 .32156]);
      | plot([xrad -x x xrad], [yrad -y y yrad]);
      | fprintf('NI Out%d', portnum);
  x_hat : S-Function  Priority=1  FunctionName=NIVeriStandIO  Parameters=width dtype portnum stime stype btype  SFunctionDeploymentMode=off  EnableBusSupport=off  mask(NI VeriStand Outport){portnum=1, width=-1, stime=-1, dtype=auto, stype=auto, btype=0}
      mask prompts: portnum "Port number:"; width "Port dimensions (-1 for dynamically sized):"; stime "Sample time (-1 for inherited):"; dtype "Data type:"; stype "Signal type:"; btype "Block type:"
      mask help: Use this outport on any level of nested subsystems to allow NI VeriStand software to map signals to it.
      mask init:
      | NIVeriStandIO_init;
      settings: CopyFcn=NIVeriStand_MDL_functions('', 'IO_copy');  DeleteFcn=NIVeriStand_MDL_functions('', 'IO_delete');  MoveFcn=set_param(gcb, 'Mask', 'on');
      mask Callback portnum: NIVeriStand_MDL_functions('', 'IO_setportnum');
      mask TypeOptions dtype: auto | double | single | int8 | uint8 | int16 | uint16 | int32 | uint32 | boolean
      mask Callback dtype: NIVeriStand_MDL_functions('', 'IO_booleansignal');
      mask TypeOptions stype: auto | real | complex
      mask Display:
      | patch([-x x], [-y y], [.90980 .81960 .32156]);
      | plot([xrad -x x xrad], [yrad -y y yrad]);
      | fprintf('NI Out%d', portnum);
  y_hat : S-Function  Priority=2  FunctionName=NIVeriStandIO  Parameters=width dtype portnum stime stype btype  SFunctionDeploymentMode=off  EnableBusSupport=off  mask(NI VeriStand Outport){portnum=2, width=-1, stime=-1, dtype=auto, stype=auto, btype=0}
      mask prompts: portnum "Port number:"; width "Port dimensions (-1 for dynamically sized):"; stime "Sample time (-1 for inherited):"; dtype "Data type:"; stype "Signal type:"; btype "Block type:"
      mask help: Use this outport on any level of nested subsystems to allow NI VeriStand software to map signals to it.
      mask init:
      | NIVeriStandIO_init;
      settings: CopyFcn=NIVeriStand_MDL_functions('', 'IO_copy');  DeleteFcn=NIVeriStand_MDL_functions('', 'IO_delete');  MoveFcn=set_param(gcb, 'Mask', 'on');
      mask Callback portnum: NIVeriStand_MDL_functions('', 'IO_setportnum');
      mask TypeOptions dtype: auto | double | single | int8 | uint8 | int16 | uint16 | int32 | uint32 | boolean
      mask Callback dtype: NIVeriStand_MDL_functions('', 'IO_booleansignal');
      mask TypeOptions stype: auto | real | complex
      mask Display:
      | patch([-x x], [-y y], [.90980 .81960 .32156]);
      | plot([xrad -x x xrad], [yrad -y y yrad]);
      | fprintf('NI Out%d', portnum);
  wires:
  Demux/1 -> x_hat/1
  Demux/2 -> y_hat/1
  Demux/3 -> psi_hat/1
  eta-_hat/1 -> Demux/1

== system ctrl_custom/Observer output /nu_dot_hat output ==
  nu_dot_hat : Inport
  Demux : Demux  Outputs=3
  r_dot_hat : S-Function  Priority=3  FunctionName=NIVeriStandIO  Parameters=width dtype portnum stime stype btype  SFunctionDeploymentMode=off  EnableBusSupport=off  mask(NI VeriStand Outport){portnum=3, width=-1, stime=-1, dtype=auto, stype=auto, btype=0}
      mask prompts: portnum "Port number:"; width "Port dimensions (-1 for dynamically sized):"; stime "Sample time (-1 for inherited):"; dtype "Data type:"; stype "Signal type:"; btype "Block type:"
      mask help: Use this outport on any level of nested subsystems to allow NI VeriStand software to map signals to it.
      mask init:
      | NIVeriStandIO_init;
      settings: CopyFcn=NIVeriStand_MDL_functions('', 'IO_copy');  DeleteFcn=NIVeriStand_MDL_functions('', 'IO_delete');  MoveFcn=set_param(gcb, 'Mask', 'on');
      mask Callback portnum: NIVeriStand_MDL_functions('', 'IO_setportnum');
      mask TypeOptions dtype: auto | double | single | int8 | uint8 | int16 | uint16 | int32 | uint32 | boolean
      mask Callback dtype: NIVeriStand_MDL_functions('', 'IO_booleansignal');
      mask TypeOptions stype: auto | real | complex
      mask Display:
      | patch([-x x], [-y y], [.90980 .81960 .32156]);
      | plot([xrad -x x xrad], [yrad -y y yrad]);
      | fprintf('NI Out%d', portnum);
  u_dot_hat : S-Function  Priority=1  FunctionName=NIVeriStandIO  Parameters=width dtype portnum stime stype btype  SFunctionDeploymentMode=off  EnableBusSupport=off  mask(NI VeriStand Outport){portnum=1, width=-1, stime=-1, dtype=auto, stype=auto, btype=0}
      mask prompts: portnum "Port number:"; width "Port dimensions (-1 for dynamically sized):"; stime "Sample time (-1 for inherited):"; dtype "Data type:"; stype "Signal type:"; btype "Block type:"
      mask help: Use this outport on any level of nested subsystems to allow NI VeriStand software to map signals to it.
      mask init:
      | NIVeriStandIO_init;
      settings: CopyFcn=NIVeriStand_MDL_functions('', 'IO_copy');  DeleteFcn=NIVeriStand_MDL_functions('', 'IO_delete');  MoveFcn=set_param(gcb, 'Mask', 'on');
      mask Callback portnum: NIVeriStand_MDL_functions('', 'IO_setportnum');
      mask TypeOptions dtype: auto | double | single | int8 | uint8 | int16 | uint16 | int32 | uint32 | boolean
      mask Callback dtype: NIVeriStand_MDL_functions('', 'IO_booleansignal');
      mask TypeOptions stype: auto | real | complex
      mask Display:
      | patch([-x x], [-y y], [.90980 .81960 .32156]);
      | plot([xrad -x x xrad], [yrad -y y yrad]);
      | fprintf('NI Out%d', portnum);
  v_dot_hat : S-Function  Priority=2  FunctionName=NIVeriStandIO  Parameters=width dtype portnum stime stype btype  SFunctionDeploymentMode=off  EnableBusSupport=off  mask(NI VeriStand Outport){portnum=2, width=-1, stime=-1, dtype=auto, stype=auto, btype=0}
      mask prompts: portnum "Port number:"; width "Port dimensions (-1 for dynamically sized):"; stime "Sample time (-1 for inherited):"; dtype "Data type:"; stype "Signal type:"; btype "Block type:"
      mask help: Use this outport on any level of nested subsystems to allow NI VeriStand software to map signals to it.
      mask init:
      | NIVeriStandIO_init;
      settings: CopyFcn=NIVeriStand_MDL_functions('', 'IO_copy');  DeleteFcn=NIVeriStand_MDL_functions('', 'IO_delete');  MoveFcn=set_param(gcb, 'Mask', 'on');
      mask Callback portnum: NIVeriStand_MDL_functions('', 'IO_setportnum');
      mask TypeOptions dtype: auto | double | single | int8 | uint8 | int16 | uint16 | int32 | uint32 | boolean
      mask Callback dtype: NIVeriStand_MDL_functions('', 'IO_booleansignal');
      mask TypeOptions stype: auto | real | complex
      mask Display:
      | patch([-x x], [-y y], [.90980 .81960 .32156]);
      | plot([xrad -x x xrad], [yrad -y y yrad]);
      | fprintf('NI Out%d', portnum);
  wires:
  Demux/1 -> u_dot_hat/1
  Demux/2 -> v_dot_hat/1
  Demux/3 -> r_dot_hat/1
  nu_dot_hat/1 -> Demux/1

== system ctrl_custom/Observer output /nu_hat output ==
  nu_hat : Inport
  Demux : Demux  Outputs=3
  r_hat : S-Function  Priority=3  FunctionName=NIVeriStandIO  Parameters=width dtype portnum stime stype btype  SFunctionDeploymentMode=off  EnableBusSupport=off  mask(NI VeriStand Outport){portnum=3, width=-1, stime=-1, dtype=auto, stype=auto, btype=0}
      mask prompts: portnum "Port number:"; width "Port dimensions (-1 for dynamically sized):"; stime "Sample time (-1 for inherited):"; dtype "Data type:"; stype "Signal type:"; btype "Block type:"
      mask help: Use this outport on any level of nested subsystems to allow NI VeriStand software to map signals to it.
      mask init:
      | NIVeriStandIO_init;
      settings: CopyFcn=NIVeriStand_MDL_functions('', 'IO_copy');  DeleteFcn=NIVeriStand_MDL_functions('', 'IO_delete');  MoveFcn=set_param(gcb, 'Mask', 'on');
      mask Callback portnum: NIVeriStand_MDL_functions('', 'IO_setportnum');
      mask TypeOptions dtype: auto | double | single | int8 | uint8 | int16 | uint16 | int32 | uint32 | boolean
      mask Callback dtype: NIVeriStand_MDL_functions('', 'IO_booleansignal');
      mask TypeOptions stype: auto | real | complex
      mask Display:
      | patch([-x x], [-y y], [.90980 .81960 .32156]);
      | plot([xrad -x x xrad], [yrad -y y yrad]);
      | fprintf('NI Out%d', portnum);
  u_hat : S-Function  Priority=1  FunctionName=NIVeriStandIO  Parameters=width dtype portnum stime stype btype  SFunctionDeploymentMode=off  EnableBusSupport=off  mask(NI VeriStand Outport){portnum=1, width=-1, stime=-1, dtype=auto, stype=auto, btype=0}
      mask prompts: portnum "Port number:"; width "Port dimensions (-1 for dynamically sized):"; stime "Sample time (-1 for inherited):"; dtype "Data type:"; stype "Signal type:"; btype "Block type:"
      mask help: Use this outport on any level of nested subsystems to allow NI VeriStand software to map signals to it.
      mask init:
      | NIVeriStandIO_init;
      settings: CopyFcn=NIVeriStand_MDL_functions('', 'IO_copy');  DeleteFcn=NIVeriStand_MDL_functions('', 'IO_delete');  MoveFcn=set_param(gcb, 'Mask', 'on');
      mask Callback portnum: NIVeriStand_MDL_functions('', 'IO_setportnum');
      mask TypeOptions dtype: auto | double | single | int8 | uint8 | int16 | uint16 | int32 | uint32 | boolean
      mask Callback dtype: NIVeriStand_MDL_functions('', 'IO_booleansignal');
      mask TypeOptions stype: auto | real | complex
      mask Display:
      | patch([-x x], [-y y], [.90980 .81960 .32156]);
      | plot([xrad -x x xrad], [yrad -y y yrad]);
      | fprintf('NI Out%d', portnum);
  v_hat : S-Function  Priority=2  FunctionName=NIVeriStandIO  Parameters=width dtype portnum stime stype btype  SFunctionDeploymentMode=off  EnableBusSupport=off  mask(NI VeriStand Outport){portnum=2, width=-1, stime=-1, dtype=auto, stype=auto, btype=0}
      mask prompts: portnum "Port number:"; width "Port dimensions (-1 for dynamically sized):"; stime "Sample time (-1 for inherited):"; dtype "Data type:"; stype "Signal type:"; btype "Block type:"
      mask help: Use this outport on any level of nested subsystems to allow NI VeriStand software to map signals to it.
      mask init:
      | NIVeriStandIO_init;
      settings: CopyFcn=NIVeriStand_MDL_functions('', 'IO_copy');  DeleteFcn=NIVeriStand_MDL_functions('', 'IO_delete');  MoveFcn=set_param(gcb, 'Mask', 'on');
      mask Callback portnum: NIVeriStand_MDL_functions('', 'IO_setportnum');
      mask TypeOptions dtype: auto | double | single | int8 | uint8 | int16 | uint16 | int32 | uint32 | boolean
      mask Callback dtype: NIVeriStand_MDL_functions('', 'IO_booleansignal');
      mask TypeOptions stype: auto | real | complex
      mask Display:
      | patch([-x x], [-y y], [.90980 .81960 .32156]);
      | plot([xrad -x x xrad], [yrad -y y yrad]);
      | fprintf('NI Out%d', portnum);
  wires:
  Demux/1 -> u_hat/1
  Demux/2 -> v_hat/1
  Demux/3 -> r_hat/1
  nu_hat/1 -> Demux/1

== system ctrl_custom/Thrust allocation/Optimal angle path and constraints on rotation speed ==
  Desired Angle : Inport  Partition=on  PartitionDimension=1  PartitionWidth=1
  "initial angle " : Inport  Port=2  Partition=on  PartitionDimension=1  PartitionWidth=1
  reset : Inport  Port=3  Partition=on  PartitionDimension=1  PartitionWidth=1
  Degrees to Radians : simulink_extras/Transformations/Degrees to Radians
  Delay : Delay  DelayLength=1  InitialCondition=0
  Discrete-Time Integrator : DiscreteIntegrator  ExternalReset=either  InitialConditionSource=external  InitialConditionSetting=State (most efficient)  SampleTime=0.01  ICPrevOutput=DiscIntNeverNeededParam  ICPrevScaledInput=DiscIntNeverNeededParam
  Ensuring angle is [-pi pi] : MATLAB Function  TreatAsAtomicUnit=on
  For Each : ForEach  DisableCoverage=on  IndexMode=One-based
  MATLAB Function1 : MATLAB Function  TreatAsAtomicUnit=on
  Max Rotation Rate : Saturate  UpperLimit=Max_rotation  LowerLimit=-Max_rotation
  commanded Angle : Outport  ConcatenationDimension=1
  wires:
  Degrees to Radians/1 -> Ensuring angle is [-pi pi]/1(angle)
  Ensuring angle is [-pi pi]/1(y) -> commanded Angle/1
  Discrete-Time Integrator/1 -> Degrees to Radians/1, Delay/1  "angle"
  "initial angle "/1 -> Discrete-Time Integrator/3
  Max Rotation Rate/1 -> Discrete-Time Integrator/1
  MATLAB Function1/1(psi_D) -> Max Rotation Rate/1
  Desired Angle/1 -> MATLAB Function1/1(desired)
  reset/1 -> Discrete-Time Integrator/2
  Delay/1 -> MATLAB Function1/2(actual)

== system ctrl_custom/Thruster control /Subsystem1 ==
  Calculated angles : Inport
  Demux : Demux  Outputs=6
  Mux : Mux  Inputs=6
  Saturation {1..6} (6 alike) : Saturate  UpperLimit=pi  LowerLimit=-pi
  Commanded angles : Outport
  wires:
  Calculated angles/1 -> Demux/1
  Demux/1 -> Saturation 1/1
  Demux/2 -> Saturation 2/1
  Demux/3 -> Saturation 3/1
  Demux/4 -> Saturation 4/1
  Demux/5 -> Saturation 5/1
  Demux/6 -> Saturation 6/1
  Mux/1 -> Commanded angles/1
  Saturation 1/1 -> Mux/1
  Saturation 6/1 -> Mux/6
  Saturation 5/1 -> Mux/5
  Saturation 2/1 -> Mux/2
  Saturation 3/1 -> Mux/3
  Saturation 4/1 -> Mux/4
